simulink model "Controle_Gimbal"  (R2026a)
settings: Solver=VariableStepAuto  StopTime=10
libraries: slpidlib x1, simulink x1
settings Model: LastModifiedBy=goncalo

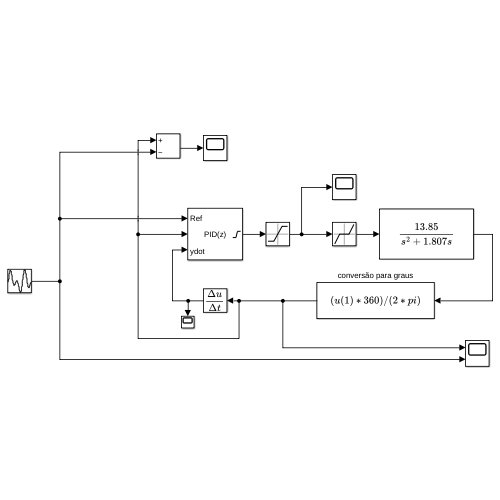
[thumbnail: Simulink's stored preview of the top-level diagram]
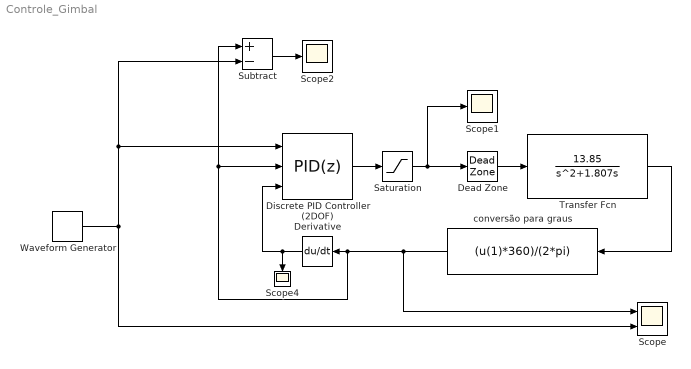
== system Controle_Gimbal ==
  Dead Zone : DeadZone  LowerValue=-0.3  UpperValue=0.3
  Derivative : Derivative
  Discrete PID Controller (2DOF) : slpidlib/PID Controller (2DOF)  Controller=PID  Form=Parallel  TimeDomain=Discrete-time  UseExternalTs=off  SampleTime=1e-4  IntegratorMethod=Forward Euler  FilterMethod=Forward Euler  ControllerParametersSource=internal  P=102.583884229566  I=891.418265022268  UseKiTs=off  D=1.45834239009198  UseExternalDerivativeSource=on  N=17380.9216379471  UseFilter=on  b=1  c=1  TunerSelectOption=Transfer Function Based (PID Tuner App)  InitialConditionSource=internal  InitialConditionForIntegrator=0  InitialConditionForFilter=0  DifferentiatorICPrevScaledInput=0  ExternalReset=none  TrackingMode=off  Kt=1  LimitOutput=on  SatLimitsSource=internal  UpperSaturationLimit=8  LowerSaturationLimit=-8  LinearizeAsGain=off  AntiWindupMode=clamping  Kb=1  LimitIntegrator=off  UpperIntegratorSaturationLimit=8  LowerIntegratorSaturationLimit=8  POutMin=[]  POutMax=[]  IOutMin=[]  IOutMax=[]  DOutMin=[]  DOutMax=[]  NOutMin=[]  NOutMax=[]  bOutMin=[]  bOutMax=[]  cOutMin=[]  cOutMax=[]  SumOutMin=[]  SumOutMax=[]  SaturationOutMin=[]  SaturationOutMax=[]  PParamMin=[]  PParamMax=[]  IParamMin=[]  IParamMax=[]  DParamMin=[]  DParamMax=[]  NParamMin=[]  NParamMax=[]  bParamMin=[]  bParamMax=[]  cParamMin=[]  cParamMax=[]  KbParamMin=[]  KbParamMax=[]  KtParamMin=[]  KtParamMax=[]  KbOutMin=[]  KbOutMax=[]  KtOutMin=[]  KtOutMax=[]  IntegratorOutMin=[]  IntegratorOutMax=[]  FilterOutMin=[]  FilterOutMax=[]  SumI1OutMin=[]  SumI1OutMax=[]  SumI2OutMin=[]  SumI2OutMax=[]  SumI3OutMin=[]  SumI3OutMax=[]  SumI4OutMin=[]  SumI4OutMax=[]  SumDOutMin=[]  SumDOutMax=[]  Sum1OutMin=[]  Sum1OutMax=[]  Sum2OutMin=[]  Sum2OutMax=[]  Sum3OutMin=[]  Sum3OutMax=[]  DifferentiatorOutMin=[]  DifferentiatorOutMax=[]  FilterDiffOutCoefMin=[]  FilterDiffOutCoefMax=[]  ReciprocalOutMin=[]  ReciprocalOutMax=[]  SumDenOutMin=[]  SumDenOutMax=[]  SumNumOutMin=[]  SumNumOutMax=[]  DivideOutMin=[]  DivideOutMax=[]  UdiffTsProdOutMin=[]  UdiffTsProdOutMax=[]  NTsProdOutMin=[]  NTsProdOutMax=[]  UintegralTsProdOutMin=[]  UintegralTsProdOutMax=[]  UngainTsProdOutMin=[]  UngainTsProdOutMax=[]  ClampingZeroOutDataTypeStr=Inherit: Inherit via back propagation  ClampingZeroOutMin=[]  ClampingZeroOutMax=[]  FilterDenConstantOutDataTypeStr=Inherit: Inherit via back propagation  FilterDenConstantOutMin=[]  FilterDenConstantOutMax=[]  PCopyOutDataTypeStr=Inherit: Inherit via back propagation  PCopyOutMin=[]  PCopyOutMax=[]  NCopyOutDataTypeStr=Inherit: Inherit via back propagation  NCopyOutMin=[]  NCopyOutMax=[]  IntegratorContinuousStateAttributes=''  IntegratorStateMustResolveToSignalObject=off  IntegratorRTWStateStorageClass=Auto  FilterContinuousStateAttributes=''  FilterStateMustResolveToSignalObject=off  FilterRTWStateStorageClass=Auto  ParallelPVariant=InternalParameters  IdealPVariant=Disabled  IVariant=InternalParameters  DVariant=InternalParameters  bVariant=InternalParameters  cVariant=Disabled  IntegratorVariant=Discrete  SatVariant=Enabled  AWVariant=DiscClampingParallel  PCopyVariant=Disabled  TRVariant=Disabled  FdbkBlocksVariant=Forward  IdealPFdbkVariant=Disabled  SatFdbkVariant=Disabled  DerivativeFilterVariant=ForwardEulerFilterOnly  NVariant=InternalParameters  NCopyVariant=Disabled  FilterICVariant=InternalICsFilter  IntegratorICVariant=InternalICs  ExternalResetVariant=Disabled  TRSumVariant=Passthrough  SumFdbkVariant=Disabled  SumVariant=Sum_PID  TsampFilterVariant=InternalTs  TsampNgainVariant=Passthrough  TsampIntegralVariant=Disabled_SignalSpec  ExternalSaturationOutDataTypeStr=Inherit: Same as second input  DerivativeSourceVariant=ExternalYdot  PreIntVariant=InternalPreInt
      settings: LibrarySourceBlock=simulink/Discrete/Discrete PID Controller (2DOF)
  Saturation : Saturate  UpperLimit=8  LowerLimit=-8
  Scope : Scope  NumInputPorts=2
      settings: ActiveDisplayYMinimum=-0.78835421559876373  ActiveDisplayYMaximum=13.067924709738609
  Scope1 : Scope
  Scope2 : Scope
      settings: ActiveDisplayYMinimum=-0.11653760783668012  ActiveDisplayYMaximum=0.11651791326024787  DataLoggingVariableName=ScopeData2
  Scope4 : Scope
      settings: ActiveDisplayYMinimum=-3548.7827253592955  ActiveDisplayYMaximum=3767.6650887867236  DataLoggingVariableName=ScopeData4
  Subtract : Sum  Inputs=+-
  Transfer Fcn : TransferFcn  Numerator=[13.85]  Denominator=[1 1.807 0]
  Waveform Generator : simulink/Sources/Waveform Generator  OutMin=[]  OutMax=[]  OutDataTypeStr=double  SelectedSignal=2  Signals=sin(2,2,0)#step(1,0,10)  BlockNames=MultiportSwitch_e3c6503dd082402#MultiportSwitch_1ec28bbcf34b4b6  SampleTime=0.033
  conversão para graus : Fcn  Expr=(u(1)*360)/(2*pi)
  wires:
  Saturation/1 -> Scope1/1, Dead Zone/1
  Subtract/1 -> Scope2/1
  Dead Zone/1 -> Transfer Fcn/1
  Discrete PID Controller (2DOF)/1 -> Saturation/1
  Derivative/1 -> Discrete PID Controller (2DOF)/3, Scope4/1
  conversão para graus/1 -> Subtract/1, Discrete PID Controller (2DOF)/2, Derivative/1, Scope/1
  Waveform Generator/1 -> Discrete PID Controller (2DOF)/1, Subtract/2, Scope/2
  Transfer Fcn/1 -> conversão para graus/1
